simulink model "MicroGrid_Trifasico"  (R2017a)
settings: Solver=VariableStepAuto  StartTime=0.0  StopTime=.2  RelTol=1e-3
undefined symbols (not defined in the file or in its folder): st_time3
libraries: fl_lib x59, nesl_utility x25, powerlib_meascontrol x6, elec_lib x4
settings Model: Creator=erich  LastModifiedBy=erich

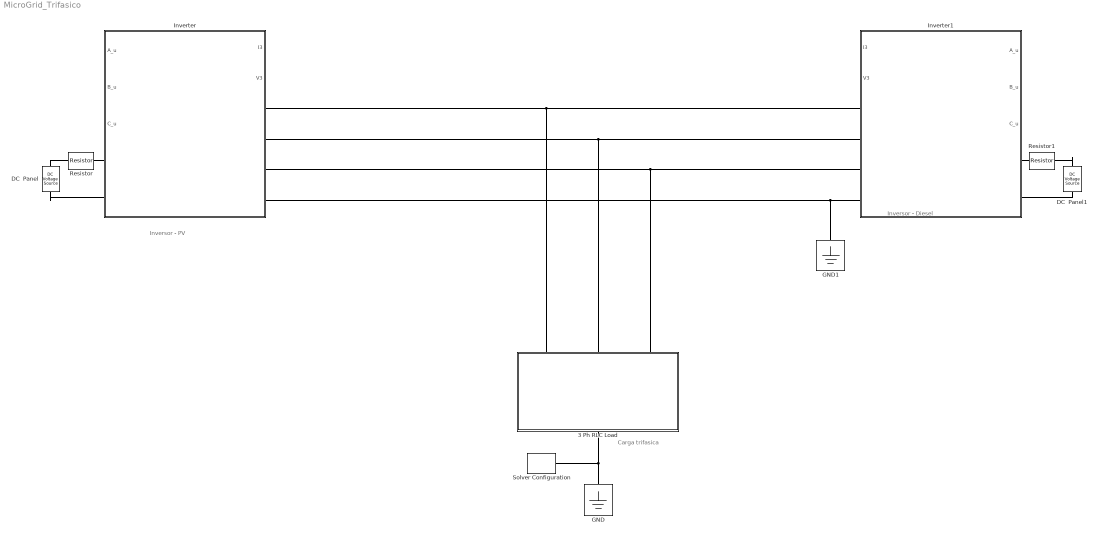
== system MicroGrid_Trifasico ==
  note: Carga trifasica
  note: Inversor - PV
  note: Inversor - Diesel
  3 Ph RLC Load : Subsystem
      mask Display:
      | port_label('lconn', 1, 'GND')
      | 
      | port_label('rconn', 1, 'Z_1', 'texmode', 'on')
      | port_label('rconn', 2, 'Z_2', 'texmode', 'on')
      | port_label('rconn', 3, 'Z_3', 'texmode', 'on')
      | 
      | plot([.15 .25], [.4 .4])
      | plot([.15 .25], [.48 .48])
      | plot([.20 .20], [.48 .6])
      | plot([.20 .20], [.4 .28])
      | 
      | plot(.43+abs(sin(200*[.2:.001:.5]/(2*pi))/15), [.2:.001:.5]+.1)
      | plot([.438 .438], [.2 .3])
      | plot([.438 .438], [.6 .7])
      | 
      | 
      | plot([.67 .73], [.6 .6])
      | plot([.67 .73], [.3 .3])
      | 
      | plot([.7 .7], [.2 .3])
      | plot([.7 .7], [.6 .7])
      | 
      | plot([.67 .67], [.6 .3])
      | plot([.73 .73], [.6 .3])
  DC  Panel : elec_lib/Additional Components/SPICE-Compatible Components/Sources/DC Voltage Source  DC=340 V
      settings: SourceProductName=Simscape Electronics  SourceProductBaseCode=SN
  DC  Panel1 : elec_lib/Additional Components/SPICE-Compatible Components/Sources/DC Voltage Source  DC=340 V
      settings: SourceProductName=Simscape Electronics  SourceProductBaseCode=SN
  GND : fl_lib/Electrical/Electrical Elements/Electrical Reference
  GND1 : fl_lib/Electrical/Electrical Elements/Electrical Reference
  Inverter : Subsystem
      mask Display:
      | port_label('input', 1, 'A_u')
      | port_label('input', 2, 'B_u')
      | port_label('input', 3, 'C_u')
      | 
      | port_label('lconn', 1, 'DC +')
      | port_label('lconn', 2, 'DC -')
      | 
      | 
      | port_label('rconn', 1, 'A')
      | port_label('rconn', 2, 'B')
      | port_label('rconn', 3, 'C')
      | 
      | port_label('output', 1, 'I_{3\Phi}', 'texmode', 'on')
      | port_label('output', 2, 'V_{3\Phi}', 'texmode', 'on')
      | 
      | plot([0.1 .9], [0.1 .9])
      | plot([0.2 .4], [.7 .7])
      | plot([0.2 .24], [.65 .65])
      | plot([0.28 .32], [.65 .65])
      | plot([0.36 .40], [.65 .65])
      | 
      | plot([.5:.01:.7], .25+sin(30*[.2:.01:.4])/10)
  Inverter1 : Subsystem
      mask Display:
      | port_label('input', 1, 'A_u')
      | port_label('input', 2, 'B_u')
      | port_label('input', 3, 'C_u')
      | 
      | port_label('lconn', 1, 'DC +')
      | port_label('lconn', 2, 'DC -')
      | 
      | 
      | port_label('rconn', 1, 'A')
      | port_label('rconn', 2, 'B')
      | port_label('rconn', 3, 'C')
      | 
      | port_label('output', 1, 'I_{3\Phi}', 'texmode', 'on')
      | port_label('output', 2, 'V_{3\Phi}', 'texmode', 'on')
      | 
      | plot([0.1 .9], [0.1 .9])
      | plot([0.2 .4], [.7 .7])
      | plot([0.2 .24], [.65 .65])
      | plot([0.28 .32], [.65 .65])
      | plot([0.36 .40], [.65 .65])
      | 
      | plot([.5:.01:.7], .25+sin(30*[.2:.01:.4])/10)
  Resistor : elec_lib/Passive Devices/Resistor  R=.01 Ohm  R_tol=5  enable_R_tol=0  tol_distribution=1  nSigma=4  enable_operating_limits=0  operating_limit_action=2  max_working_voltage=100 V  power_rating=1 W  enable_faults=0  fault_action=1  R_faulted=inf Ohm  enable_temporal_fault=0  t_fault=1 s  enable_behavioral_fault=0  max_permissible_current=1 A  t_fail_on_current=1 s  noise_mode=0  sample_time=1e-3 s  repeatability=1  auto_seed=1274213173  user_seed=0  Tdevice=25 degC  alpha=3.93e-3 1/K  Tmeas=25 degC  thermal_mass=100 J/K  power_derating_T1=70 degC  power_derating_T2=155 degC  operating_temperature_range_vec=[-50.0, 150.0] degC  temperature_specify=off  temperature_priority=High  temperature=298.15 K  temperature_nominal_specify=off  temperature_nominal_unit=K  temperature_nominal_value=1
  Resistor1 : elec_lib/Passive Devices/Resistor  R=1 Ohm  R_tol=5  enable_R_tol=0  tol_distribution=1  nSigma=4  enable_operating_limits=0  operating_limit_action=2  max_working_voltage=100 V  power_rating=1 W  enable_faults=0  fault_action=1  R_faulted=inf Ohm  enable_temporal_fault=0  t_fault=1 s  enable_behavioral_fault=0  max_permissible_current=1 A  t_fail_on_current=1 s  noise_mode=0  sample_time=1e-3 s  repeatability=1  auto_seed=306855934  user_seed=0  Tdevice=25 degC  alpha=3.93e-3 1/K  Tmeas=25 degC  thermal_mass=100 J/K  power_derating_T1=70 degC  power_derating_T2=155 degC  operating_temperature_range_vec=[-50.0, 150.0] degC  temperature_specify=off  temperature_priority=High  temperature=298.15 K  temperature_nominal_specify=off  temperature_nominal_unit=K  temperature_nominal_value=1
  Solver Configuration : nesl_utility/Solver Configuration  PhysicalDomain=network_engine_domain  SubClassName=solver  LeftPortType=input  RightPortType=generic  Accelerate=off  Tones=[]  Harmonics=[]  SimulateNoise=off  Profile=off  UseLocalSampling=off  EnableSwitchedLinearOptims=on  FrequencyDomain=off  UseCCode=off  RelTol=0.001  AbsTol=1e-06  MinStep=1e-09  ToWorkspace=off  RevertToSquareIcSolve=off  NumHomotopyIterations=100  PhasorMode=off  PhasorModeNumHarmonics=1  OverrideAbsTol=off  DoDC=off  ResidualTolerance=1e-09  UseLocalSolver=on  LocalSolverChoice=NE_BACKWARD_EULER_ADVANCER  LocalSolverSampleTime=1e-6  DoFixedCost=on  MaxNonlinIter=3  MaxModeIter=2  LinearAlgebra=Sparse  DelaysMemoryBudget=1024  AutomaticFiltering=on  FilteringTimeConstant=0.001
  connections:
  3 Ph RLC Load/LConn1 -- GND/LConn1 -- Solver Configuration/RConn1
  Resistor/LConn1 -- DC  Panel/LConn1
  DC  Panel/RConn1 -- Inverter/LConn2
  Resistor/RConn1 -- Inverter/LConn1
  Inverter1/LConn2 -- DC  Panel1/LConn1
  DC  Panel1/RConn1 -- Resistor1/LConn1
  Inverter1/LConn1 -- Resistor1/RConn1
  Inverter/RConn1 -- 3 Ph RLC Load/RConn1 -- Inverter1/RConn1
  Inverter1/RConn2 -- 3 Ph RLC Load/RConn2 -- Inverter/RConn2
  Inverter1/RConn3 -- 3 Ph RLC Load/RConn3 -- Inverter/RConn3
  Inverter1/RConn4 -- GND1/LConn1 -- Inverter/RConn4

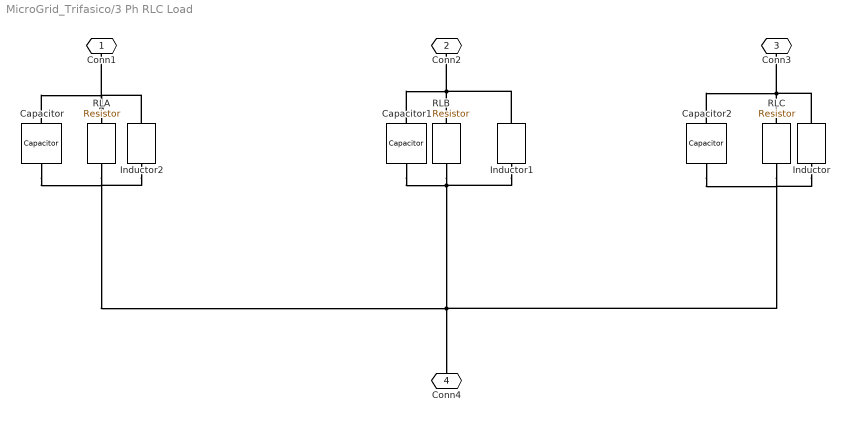
== system MicroGrid_Trifasico/3 Ph RLC Load ==
  Capacitor : fl_lib/Electrical/Electrical Elements/Capacitor  c=100e-6 uF  r=1e-6 Ohm  g=0 1/Ohm  i_specify=off  i_priority=None  i=0 A  i_nominal_specify=off  i_nominal_unit=A  i_nominal_value=1  v_specify=off  v_priority=None  v=0 V  v_nominal_specify=off  v_nominal_unit=V  v_nominal_value=1  vc_specify=off  vc_priority=High  vc=0 V  vc_nominal_specify=off  vc_nominal_unit=V  vc_nominal_value=1
  Capacitor1 : fl_lib/Electrical/Electrical Elements/Capacitor  c=100e-6 uF  r=1e-6 Ohm  g=0 1/Ohm  i_specify=off  i_priority=None  i=0 A  i_nominal_specify=off  i_nominal_unit=A  i_nominal_value=1  v_specify=off  v_priority=None  v=0 V  v_nominal_specify=off  v_nominal_unit=V  v_nominal_value=1  vc_specify=off  vc_priority=High  vc=0 V  vc_nominal_specify=off  vc_nominal_unit=V  vc_nominal_value=1
  Capacitor2 : fl_lib/Electrical/Electrical Elements/Capacitor  c=100e-6 uF  r=1e-6 Ohm  g=0 1/Ohm  i_specify=off  i_priority=None  i=0 A  i_nominal_specify=off  i_nominal_unit=A  i_nominal_value=1  v_specify=off  v_priority=None  v=0 V  v_nominal_specify=off  v_nominal_unit=V  v_nominal_value=1  vc_specify=off  vc_priority=High  vc=0 V  vc_nominal_specify=off  vc_nominal_unit=V  vc_nominal_value=1
  Inductor : fl_lib/Electrical/Electrical Elements/Inductor  l=5200 mH  r=0 Ohm  g=100e-9 1/Ohm  i_specify=off  i_priority=None  i=0 A  i_nominal_specify=off  i_nominal_unit=A  i_nominal_value=1  v_specify=off  v_priority=None  v=0 V  v_nominal_specify=off  v_nominal_unit=V  v_nominal_value=1  i_L_specify=off  i_L_priority=High  i_L=0 A  i_L_nominal_specify=off  i_L_nominal_unit=A  i_L_nominal_value=1
  Inductor1 : fl_lib/Electrical/Electrical Elements/Inductor  l=5200 mH  r=0 Ohm  g=100e-9 1/Ohm  i_specify=off  i_priority=None  i=0 A  i_nominal_specify=off  i_nominal_unit=A  i_nominal_value=1  v_specify=off  v_priority=None  v=0 V  v_nominal_specify=off  v_nominal_unit=V  v_nominal_value=1  i_L_specify=off  i_L_priority=High  i_L=0 A  i_L_nominal_specify=off  i_L_nominal_unit=A  i_L_nominal_value=1
  Inductor2 : fl_lib/Electrical/Electrical Elements/Inductor  l=5200 mH  r=0 Ohm  g=100e-9 1/Ohm  i_specify=off  i_priority=None  i=0 A  i_nominal_specify=off  i_nominal_unit=A  i_nominal_value=1  v_specify=off  v_priority=None  v=0 V  v_nominal_specify=off  v_nominal_unit=V  v_nominal_value=1  i_L_specify=off  i_L_priority=High  i_L=0 A  i_L_nominal_specify=off  i_L_nominal_unit=A  i_L_nominal_value=1
  RLA : fl_lib/Electrical/Electrical Elements/Resistor  R=15 Ohm  i_specify=off  i_priority=None  i=0 A  i_nominal_specify=off  i_nominal_unit=A  i_nominal_value=1  v_specify=off  v_priority=None  v=0 V  v_nominal_specify=off  v_nominal_unit=V  v_nominal_value=1
  RLB : fl_lib/Electrical/Electrical Elements/Resistor  R=15 Ohm  i_specify=off  i_priority=None  i=0 A  i_nominal_specify=off  i_nominal_unit=A  i_nominal_value=1  v_specify=off  v_priority=None  v=0 V  v_nominal_specify=off  v_nominal_unit=V  v_nominal_value=1
  RLC : fl_lib/Electrical/Electrical Elements/Resistor  R=15 Ohm  i_specify=off  i_priority=None  i=0 A  i_nominal_specify=off  i_nominal_unit=A  i_nominal_value=1  v_specify=off  v_priority=None  v=0 V  v_nominal_specify=off  v_nominal_unit=V  v_nominal_value=1
  Conn1 : PMIOPort  Port=1  Side=Right
  Conn2 : PMIOPort  Port=2  Side=Right
  Conn3 : PMIOPort  Port=3  Side=Right
  Conn4 : PMIOPort  Port=4  Side=Left
  connections:
  RLB/RConn1 -- Capacitor1/RConn1 -- Inductor1/RConn1 -- Conn4/RConn1 -- Inductor2/RConn1 -- Capacitor/RConn1 -- RLA/RConn1 -- Capacitor2/RConn1 -- Inductor/RConn1 -- RLC/RConn1
  RLA/LConn1 -- Inductor2/LConn1 -- Conn1/RConn1 -- Capacitor/LConn1
  RLC/LConn1 -- Capacitor2/LConn1 -- Conn3/RConn1 -- Inductor/LConn1
  RLB/LConn1 -- Conn2/RConn1 -- Capacitor1/LConn1 -- Inductor1/LConn1

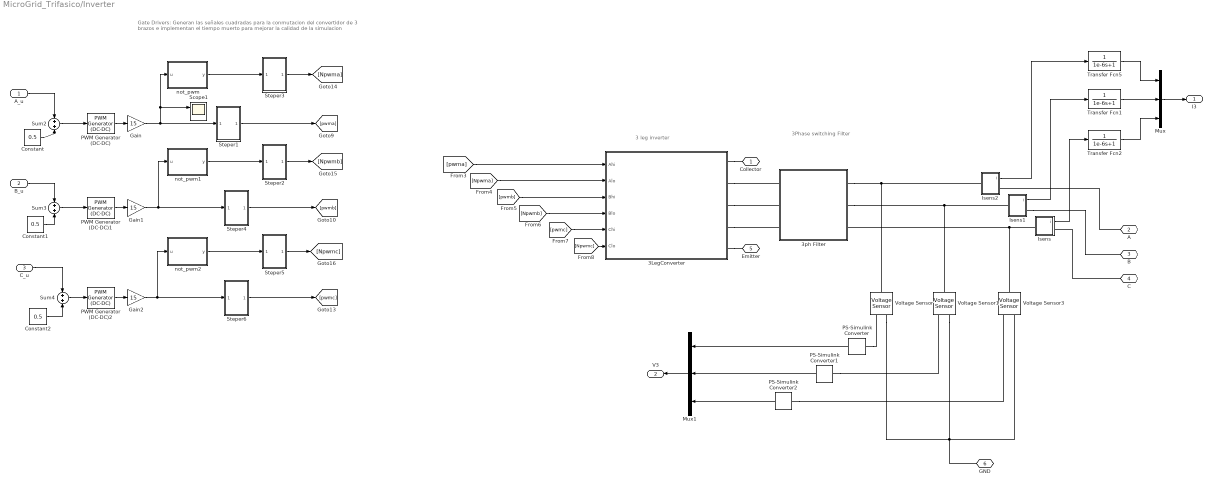
== system MicroGrid_Trifasico/Inverter ==
  note: Gate Drivers: Generan las señales cuadradas para
      | la conmutacion del convertidor de 3 brazos e implementan el
      | tiempo muerto para mejorar la calidad de la simulacion
  note: 3 leg inverter
  note: 3Phase
      | switching
      | Filter
  A_u : Inport
  B_u : Inport  Port=2
  C_u : Inport  Port=3
  3LegConverter : Subsystem
      mask Display:
      | % entradas de conmutacion del mosfet
      | port_label('input',1,'Ahi')
      | port_label('input',2,'Alo')
      | port_label('input',3,'Bhi')
      | port_label('input',4,'Blo')
      | port_label('input',5,'Chi')
      | port_label('input',6,'Clo')
      | 
      | % puertos de conexion del inversor
      | port_label('rconn',1,'Collector') % + fuente dc
      | port_label('rconn',2,'A') % fase A
      | port_label('rconn',3,'B') % fase B
      | port_label('rconn',4,'C') % fase C
      | port_label('rconn',5,'Emitter') % ref fuente dc
      | 
      | 
      | plot([.4 .4],[.35 .7])
      | plot([.2 .4],[.52 .52])
      | plot([.46 .46],[.22 .85])
      | plot([.46 .7],[.73 .73])
      | plot([.46 .7],[.32 .32])
  3ph Filter : Subsystem
      mask Display:
      | port_label('lconn', 1, 'A_{in}', 'texmode', 'on')
      | port_label('lconn', 2, 'B_{in}', 'texmode', 'on')
      | port_label('lconn', 3, 'B_{in}', 'texmode', 'on')
      | port_label('rconn', 1, 'A_{out}', 'texmode', 'on')
      | port_label('rconn', 2, 'B_{out}', 'texmode', 'on')
      | port_label('rconn', 3, 'C_{out}', 'texmode', 'on')
      | 
      | 
      | plot([.2 .5], [.7 .7])
      | plot([.5 .6], [.7 .3])
      | plot([.6 .7], [.3 .3])
      | 
      | text(.2, .8, '\fontsize{12} H(\omega)', 'texmode', 'on')
      | text(.6, .25, '\fontsize{12} \omega', 'texmode', 'on')
  Constant : Constant  Value=0.5
  Constant1 : Constant  Value=0.5
  Constant2 : Constant  Value=0.5
  Gain : Gain  Gain=15
  Gain1 : Gain  Gain=15
  Gain2 : Gain  Gain=15
  Isens : Subsystem
  Isens1 : Subsystem
  Isens2 : Subsystem
  Mux : Mux  Inputs=3
  Mux1 : Mux  Inputs=3
  PS-Simulink Converter : nesl_utility/PS-Simulink Converter  PhysicalDomain=network_engine_domain  SubClassName=ps_output  LeftPortType=input  RightPortType=output  PseudoPeriodic=off  Frequencies=[]  Unit=1  AffineConversion=off
  PS-Simulink Converter1 : nesl_utility/PS-Simulink Converter  PhysicalDomain=network_engine_domain  SubClassName=ps_output  LeftPortType=input  RightPortType=output  PseudoPeriodic=off  Frequencies=[]  Unit=1  AffineConversion=off
  PS-Simulink Converter2 : nesl_utility/PS-Simulink Converter  PhysicalDomain=network_engine_domain  SubClassName=ps_output  LeftPortType=input  RightPortType=output  PseudoPeriodic=off  Frequencies=[]  Unit=1  AffineConversion=off
  PWM Generator (DC-DC) : powerlib_meascontrol/Pulse & Signal Generators/PWM Generator (DC-DC)  Fsw=5000  Ts=0
  PWM Generator (DC-DC)1 : powerlib_meascontrol/Pulse & Signal Generators/PWM Generator (DC-DC)  Fsw=5000  Ts=0
  PWM Generator (DC-DC)2 : powerlib_meascontrol/Pulse & Signal Generators/PWM Generator (DC-DC)  Fsw=5000  Ts=0
  Scope1 : Scope  NumInputPorts=2
  Steper1 : Subsystem
  Steper2 : Subsystem
  Steper3 : Subsystem
  Steper4 : Subsystem
  Steper5 : Subsystem
  Steper6 : Subsystem
  Sum2 : Sum
  Sum3 : Sum
  Sum4 : Sum
  Transfer Fcn1 : TransferFcn  Denominator=[1e-6 1]
  Transfer Fcn2 : TransferFcn  Denominator=[1e-6 1]
  Transfer Fcn5 : TransferFcn  Denominator=[1e-6 1]
  Voltage Sensor : fl_lib/Electrical/Electrical Sensors/Voltage Sensor
  Voltage Sensor1 : fl_lib/Electrical/Electrical Sensors/Voltage Sensor
  Voltage Sensor3 : fl_lib/Electrical/Electrical Sensors/Voltage Sensor
  not_pwm : MATLAB Function  TreatAsAtomicUnit=on
  not_pwm1 : MATLAB Function  TreatAsAtomicUnit=on
  not_pwm2 : MATLAB Function  TreatAsAtomicUnit=on
  Collector : PMIOPort  Port=1  Side=Left
  A : PMIOPort  Port=2  Side=Right
  B : PMIOPort  Port=3  Side=Right
  C : PMIOPort  Port=4  Side=Right
  Emitter : PMIOPort  Port=5  Side=Left
  GND : PMIOPort  Port=6  Side=Right
  I3 : Outport
  V3 : Outport  Port=2
  wires:
  C_u/1 -> Sum4/1
  [Npwmc] -> 3LegConverter/6(Clo)
  [pwma] -> 3LegConverter/1(Ahi)
  [pwmc] -> 3LegConverter/5(Chi)
  [Npwma] -> 3LegConverter/2(Alo)
  [Npwmb] -> 3LegConverter/4(Blo)
  [pwmb] -> 3LegConverter/3(Bhi)
  Steper5/1(Out1) -> [Npwmc]
  Steper4/1(Out1) -> [pwmb]
  Gain/1 -> Steper1/1(In1), Scope1/1, not_pwm/1(u)
  not_pwm1/1(y) -> Steper2/1(In1)
  Steper3/1(Out1) -> [Npwma]
  Constant/1 -> Sum2/2
  Sum2/1 -> PWM Generator (DC-DC)/1
  Gain2/1 -> Steper6/1(In1), not_pwm2/1(u)
  Sum3/1 -> PWM Generator (DC-DC)1/1
  Steper6/1(Out1) -> [pwmc]
  Sum4/1 -> PWM Generator (DC-DC)2/1
  Gain1/1 -> Steper4/1(In1), not_pwm1/1(u)
  not_pwm2/1(y) -> Steper5/1(In1)
  Steper2/1(Out1) -> [Npwmb]
  Constant2/1 -> Sum4/2
  PWM Generator (DC-DC)1/1 -> Gain1/1
  not_pwm/1(y) -> Steper3/1(In1)
  PWM Generator (DC-DC)/1 -> Gain/1
  PWM Generator (DC-DC)2/1 -> Gain2/1
  Steper1/1(Out1) -> [pwma]
  Constant1/1 -> Sum3/2
  B_u/1 -> Sum3/1
  A_u/1 -> Sum2/1
  Isens/1(i) -> Transfer Fcn2/1
  Isens1/1(i) -> Transfer Fcn1/1
  Isens2/1(i) -> Transfer Fcn5/1
  Mux/1 -> I3/1
  Transfer Fcn1/1 -> Mux/2
  Transfer Fcn5/1 -> Mux/1
  Transfer Fcn2/1 -> Mux/3
  Mux1/1 -> V3/1
  PS-Simulink Converter/1 -> Mux1/1
  PS-Simulink Converter1/1 -> Mux1/2
  PS-Simulink Converter2/1 -> Mux1/3
  connections:
  3LegConverter/RConn5 -- Emitter/RConn1
  3LegConverter/RConn1 -- Collector/RConn1
  C/RConn1 -- Isens/RConn1
  Isens1/RConn1 -- B/RConn1
  A/RConn1 -- Isens2/RConn1
  3LegConverter/RConn2 -- 3ph Filter/LConn1
  3LegConverter/RConn3 -- 3ph Filter/LConn2
  3LegConverter/RConn4 -- 3ph Filter/LConn3
  3ph Filter/RConn1 -- Voltage Sensor/LConn1 -- Isens2/LConn1
  3ph Filter/RConn2 -- Isens1/LConn1 -- Voltage Sensor1/LConn1
  Isens/LConn1 -- Voltage Sensor3/LConn1 -- 3ph Filter/RConn3
  Voltage Sensor1/RConn2 -- Voltage Sensor3/RConn2 -- GND/RConn1 -- Voltage Sensor/RConn2
  PS-Simulink Converter1/LConn1 -- Voltage Sensor1/RConn1
  PS-Simulink Converter2/LConn1 -- Voltage Sensor3/RConn1
  PS-Simulink Converter/LConn1 -- Voltage Sensor/RConn1

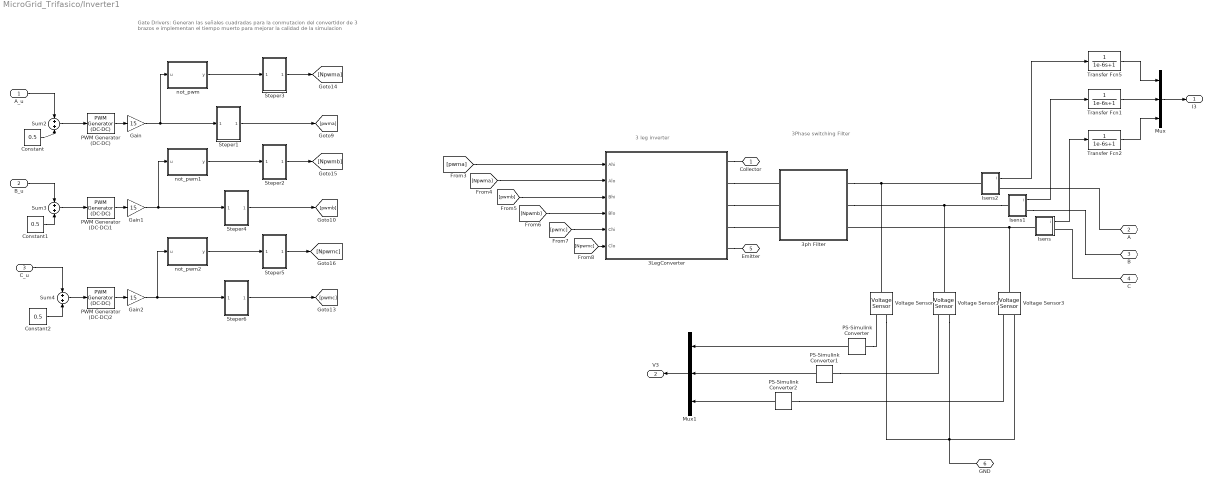
== system MicroGrid_Trifasico/Inverter1 ==
  note: 3Phase
      | switching
      | Filter
  note: 3 leg inverter
  note: Gate Drivers: Generan las señales cuadradas para
      | la conmutacion del convertidor de 3 brazos e implementan el
      | tiempo muerto para mejorar la calidad de la simulacion
  A_u : Inport
  B_u : Inport  Port=2
  C_u : Inport  Port=3
  3LegConverter : Subsystem
      mask Display:
      | % entradas de conmutacion del mosfet
      | port_label('input',1,'Ahi')
      | port_label('input',2,'Alo')
      | port_label('input',3,'Bhi')
      | port_label('input',4,'Blo')
      | port_label('input',5,'Chi')
      | port_label('input',6,'Clo')
      | 
      | % puertos de conexion del inversor
      | port_label('rconn',1,'Collector') % + fuente dc
      | port_label('rconn',2,'A') % fase A
      | port_label('rconn',3,'B') % fase B
      | port_label('rconn',4,'C') % fase C
      | port_label('rconn',5,'Emitter') % ref fuente dc
      | 
      | 
      | plot([.4 .4],[.35 .7])
      | plot([.2 .4],[.52 .52])
      | plot([.46 .46],[.22 .85])
      | plot([.46 .7],[.73 .73])
      | plot([.46 .7],[.32 .32])
  3ph Filter : Subsystem
  Constant : Constant  Value=0.5
  Constant1 : Constant  Value=0.5
  Constant2 : Constant  Value=0.5
  Gain : Gain  Gain=15
  Gain1 : Gain  Gain=15
  Gain2 : Gain  Gain=15
  Isens : Subsystem
  Isens1 : Subsystem
  Isens2 : Subsystem
  Mux : Mux  Inputs=3
  Mux1 : Mux  Inputs=3
  PS-Simulink Converter : nesl_utility/PS-Simulink Converter  PhysicalDomain=network_engine_domain  SubClassName=ps_output  LeftPortType=input  RightPortType=output  PseudoPeriodic=off  Frequencies=[]  Unit=1  AffineConversion=off
  PS-Simulink Converter1 : nesl_utility/PS-Simulink Converter  PhysicalDomain=network_engine_domain  SubClassName=ps_output  LeftPortType=input  RightPortType=output  PseudoPeriodic=off  Frequencies=[]  Unit=1  AffineConversion=off
  PS-Simulink Converter2 : nesl_utility/PS-Simulink Converter  PhysicalDomain=network_engine_domain  SubClassName=ps_output  LeftPortType=input  RightPortType=output  PseudoPeriodic=off  Frequencies=[]  Unit=1  AffineConversion=off
  PWM Generator (DC-DC) : powerlib_meascontrol/Pulse & Signal Generators/PWM Generator (DC-DC)  Fsw=5000  Ts=0
  PWM Generator (DC-DC)1 : powerlib_meascontrol/Pulse & Signal Generators/PWM Generator (DC-DC)  Fsw=5000  Ts=0
  PWM Generator (DC-DC)2 : powerlib_meascontrol/Pulse & Signal Generators/PWM Generator (DC-DC)  Fsw=5000  Ts=0
  Steper1 : Subsystem
  Steper2 : Subsystem
  Steper3 : Subsystem
  Steper4 : Subsystem
  Steper5 : Subsystem
  Steper6 : Subsystem
  Sum2 : Sum
  Sum3 : Sum
  Sum4 : Sum
  Transfer Fcn1 : TransferFcn  Denominator=[1e-6 1]
  Transfer Fcn2 : TransferFcn  Denominator=[1e-6 1]
  Transfer Fcn5 : TransferFcn  Denominator=[1e-6 1]
  Voltage Sensor : fl_lib/Electrical/Electrical Sensors/Voltage Sensor
  Voltage Sensor1 : fl_lib/Electrical/Electrical Sensors/Voltage Sensor
  Voltage Sensor3 : fl_lib/Electrical/Electrical Sensors/Voltage Sensor
  not_pwm : MATLAB Function  TreatAsAtomicUnit=on
  not_pwm1 : MATLAB Function  TreatAsAtomicUnit=on
  not_pwm2 : MATLAB Function  TreatAsAtomicUnit=on
  Collector : PMIOPort  Port=1  Side=Left
  A : PMIOPort  Port=2  Side=Right
  B : PMIOPort  Port=3  Side=Right
  C : PMIOPort  Port=4  Side=Right
  Emitter : PMIOPort  Port=5  Side=Left
  GND : PMIOPort  Port=6  Side=Right
  I3 : Outport
  V3 : Outport  Port=2
  wires:
  PS-Simulink Converter2/1 -> Mux1/3
  PS-Simulink Converter1/1 -> Mux1/2
  PS-Simulink Converter/1 -> Mux1/1
  Mux1/1 -> V3/1
  Transfer Fcn2/1 -> Mux/3
  Transfer Fcn5/1 -> Mux/1
  Transfer Fcn1/1 -> Mux/2
  Mux/1 -> I3/1
  Isens2/1(i) -> Transfer Fcn5/1
  Isens1/1(i) -> Transfer Fcn1/1
  Isens/1(i) -> Transfer Fcn2/1
  A_u/1 -> Sum2/1
  B_u/1 -> Sum3/1
  Constant1/1 -> Sum3/2
  Steper1/1(Out1) -> [pwma]
  PWM Generator (DC-DC)2/1 -> Gain2/1
  PWM Generator (DC-DC)/1 -> Gain/1
  not_pwm/1(y) -> Steper3/1(In1)
  PWM Generator (DC-DC)1/1 -> Gain1/1
  Constant2/1 -> Sum4/2
  Steper2/1(Out1) -> [Npwmb]
  not_pwm2/1(y) -> Steper5/1(In1)
  Gain1/1 -> not_pwm1/1(u), Steper4/1(In1)
  Sum4/1 -> PWM Generator (DC-DC)2/1
  Steper6/1(Out1) -> [pwmc]
  Sum3/1 -> PWM Generator (DC-DC)1/1
  Gain2/1 -> not_pwm2/1(u), Steper6/1(In1)
  Sum2/1 -> PWM Generator (DC-DC)/1
  Constant/1 -> Sum2/2
  Steper3/1(Out1) -> [Npwma]
  not_pwm1/1(y) -> Steper2/1(In1)
  Gain/1 -> not_pwm/1(u), Steper1/1(In1)
  Steper4/1(Out1) -> [pwmb]
  Steper5/1(Out1) -> [Npwmc]
  [pwmb] -> 3LegConverter/3(Bhi)
  [Npwmb] -> 3LegConverter/4(Blo)
  [Npwma] -> 3LegConverter/2(Alo)
  [pwmc] -> 3LegConverter/5(Chi)
  [pwma] -> 3LegConverter/1(Ahi)
  [Npwmc] -> 3LegConverter/6(Clo)
  C_u/1 -> Sum4/1
  connections:
  PS-Simulink Converter/LConn1 -- Voltage Sensor/RConn1
  PS-Simulink Converter2/LConn1 -- Voltage Sensor3/RConn1
  PS-Simulink Converter1/LConn1 -- Voltage Sensor1/RConn1
  Voltage Sensor3/RConn2 -- Voltage Sensor/RConn2 -- GND/RConn1 -- Voltage Sensor1/RConn2
  Voltage Sensor3/LConn1 -- 3ph Filter/RConn3 -- Isens/LConn1
  Isens1/LConn1 -- 3ph Filter/RConn2 -- Voltage Sensor1/LConn1
  Voltage Sensor/LConn1 -- 3ph Filter/RConn1 -- Isens2/LConn1
  3LegConverter/RConn4 -- 3ph Filter/LConn3
  3LegConverter/RConn3 -- 3ph Filter/LConn2
  3LegConverter/RConn2 -- 3ph Filter/LConn1
  A/RConn1 -- Isens2/RConn1
  Isens1/RConn1 -- B/RConn1
  C/RConn1 -- Isens/RConn1
  3LegConverter/RConn1 -- Collector/RConn1
  3LegConverter/RConn5 -- Emitter/RConn1

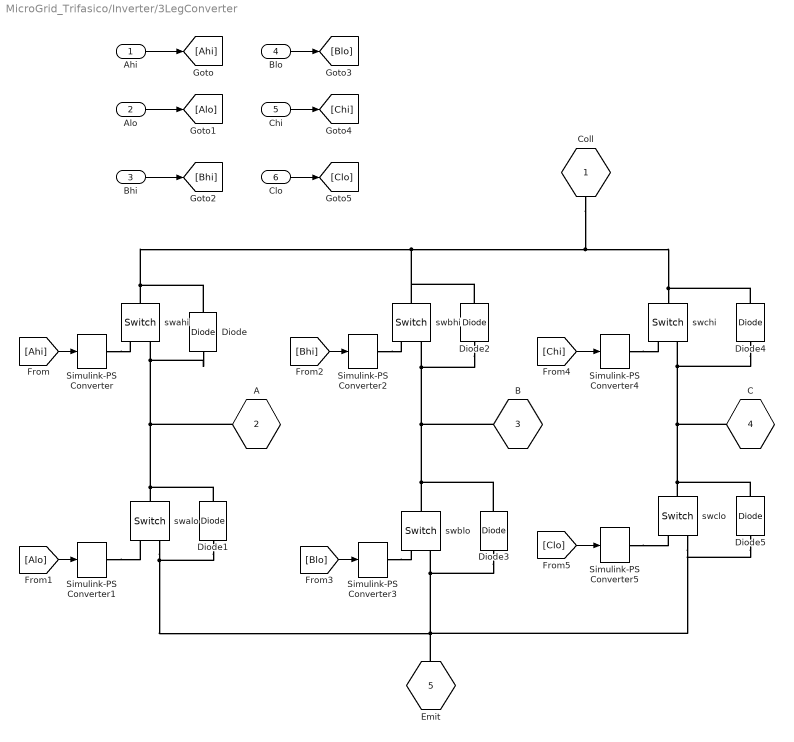
== system MicroGrid_Trifasico/Inverter/3LegConverter ==
  Ahi : Inport
  Alo : Inport  Port=2
  Bhi : Inport  Port=3
  Blo : Inport  Port=4
  Chi : Inport  Port=5
  Clo : Inport  Port=6
  Diode{,1..5} (6 alike) : fl_lib/Electrical/Electrical Elements/Diode  Vf=0.6 V  Ron=0.3 Ohm  Goff=1e-8 1/Ohm  i_specify=off  i_priority=None  i=0 A  i_nominal_specify=off  i_nominal_unit=A  i_nominal_value=1  v_specify=off  v_priority=None  v=0 V  v_nominal_specify=off  v_nominal_unit=V  v_nominal_value=1
  Simulink-PS Converter{,1..5} (6 alike) : nesl_utility/Simulink-PS Converter  PhysicalDomain=network_engine_domain  SubClassName=ps_input  LeftPortType=input  RightPortType=output  PseudoPeriodic=off  Frequencies=[]  NoiseDistribution=none  NoiseParameters=[]  Unit=1  AffineConversion=off  FilteringAndDerivatives=zero  SimscapeFilterOrder=1  InputFilterTimeConstant=0.001  UdotUserProvided=1
  swahi : fl_lib/Electrical/Electrical Elements/Switch  R_closed=0.01 Ohm  G_open=1e-8 1/Ohm  Threshold=2  i_specify=off  i_priority=None  i=0 A  i_nominal_specify=off  i_nominal_unit=A  i_nominal_value=1  v_specify=off  v_priority=None  v=0 V  v_nominal_specify=off  v_nominal_unit=V  v_nominal_value=1
      settings: SourceProductName=Simscape
  swalo : fl_lib/Electrical/Electrical Elements/Switch  R_closed=0.01 Ohm  G_open=1e-8 1/Ohm  Threshold=2  i_specify=off  i_priority=None  i=0 A  i_nominal_specify=off  i_nominal_unit=A  i_nominal_value=1  v_specify=off  v_priority=None  v=0 V  v_nominal_specify=off  v_nominal_unit=V  v_nominal_value=1
      settings: SourceProductName=Simscape
  swbhi : fl_lib/Electrical/Electrical Elements/Switch  R_closed=0.01 Ohm  G_open=1e-8 1/Ohm  Threshold=2  i_specify=off  i_priority=None  i=0 A  i_nominal_specify=off  i_nominal_unit=A  i_nominal_value=1  v_specify=off  v_priority=None  v=0 V  v_nominal_specify=off  v_nominal_unit=V  v_nominal_value=1
      settings: SourceProductName=Simscape
  swblo : fl_lib/Electrical/Electrical Elements/Switch  R_closed=0.01 Ohm  G_open=1e-8 1/Ohm  Threshold=2  i_specify=off  i_priority=None  i=0 A  i_nominal_specify=off  i_nominal_unit=A  i_nominal_value=1  v_specify=off  v_priority=None  v=0 V  v_nominal_specify=off  v_nominal_unit=V  v_nominal_value=1
      settings: SourceProductName=Simscape
  swchi : fl_lib/Electrical/Electrical Elements/Switch  R_closed=0.01 Ohm  G_open=1e-8 1/Ohm  Threshold=2  i_specify=off  i_priority=None  i=0 A  i_nominal_specify=off  i_nominal_unit=A  i_nominal_value=1  v_specify=off  v_priority=None  v=0 V  v_nominal_specify=off  v_nominal_unit=V  v_nominal_value=1
      settings: SourceProductName=Simscape
  swclo : fl_lib/Electrical/Electrical Elements/Switch  R_closed=0.01 Ohm  G_open=1e-8 1/Ohm  Threshold=2  i_specify=off  i_priority=None  i=0 A  i_nominal_specify=off  i_nominal_unit=A  i_nominal_value=1  v_specify=off  v_priority=None  v=0 V  v_nominal_specify=off  v_nominal_unit=V  v_nominal_value=1
      settings: SourceProductName=Simscape
  Coll : PMIOPort  Port=1  Side=Right
  A : PMIOPort  Port=2  Side=Right
  B : PMIOPort  Port=3  Side=Right
  C : PMIOPort  Port=4  Side=Right
  Emit : PMIOPort  Port=5  Side=Right
  wires:
  [Alo] -> Simulink-PS Converter1/1
  [Ahi] -> Simulink-PS Converter/1
  Clo/1 -> [Clo]
  Alo/1 -> [Alo]
  [Blo] -> Simulink-PS Converter3/1
  [Clo] -> Simulink-PS Converter5/1
  Bhi/1 -> [Bhi]
  [Bhi] -> Simulink-PS Converter2/1
  Ahi/1 -> [Ahi]
  [Chi] -> Simulink-PS Converter4/1
  Blo/1 -> [Blo]
  Chi/1 -> [Chi]
  connections:
  swalo/RConn2 -- Diode3/LConn1 -- swblo/RConn2 -- Emit/RConn1 -- Diode5/LConn1 -- swclo/RConn2 -- Diode1/LConn1
  Simulink-PS Converter4/RConn1 -- swchi/RConn1
  Simulink-PS Converter5/RConn1 -- swclo/RConn1
  Simulink-PS Converter/RConn1 -- swahi/RConn1
  swblo/LConn1 -- Diode3/RConn1 -- B/RConn1 -- Diode2/LConn1 -- swbhi/RConn2
  Simulink-PS Converter3/RConn1 -- swblo/RConn1
  Simulink-PS Converter2/RConn1 -- swbhi/RConn1
  Simulink-PS Converter1/RConn1 -- swalo/RConn1
  swalo/LConn1 -- A/RConn1 -- Diode/LConn1 -- swahi/RConn2 -- Diode1/RConn1
  swahi/LConn1 -- Diode/RConn1 -- Diode2/RConn1 -- swbhi/LConn1 -- Coll/RConn1 -- Diode4/RConn1 -- swchi/LConn1
  swclo/LConn1 -- Diode5/RConn1 -- C/RConn1 -- Diode4/LConn1 -- swchi/RConn2

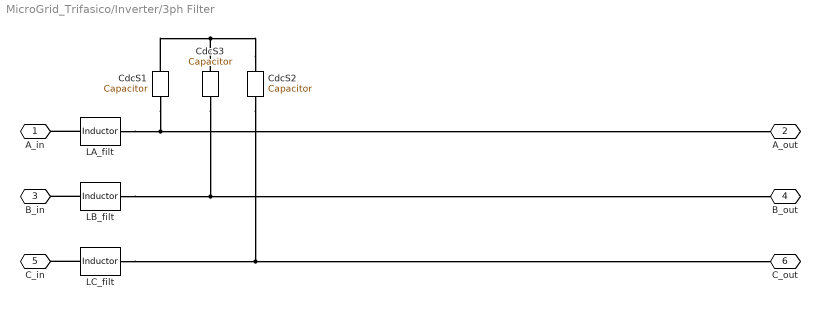
== system MicroGrid_Trifasico/Inverter/3ph Filter ==
  CdcS1 : fl_lib/Electrical/Electrical Elements/Capacitor  c=3.5 uF  r=1e-6 Ohm  g=0 1/Ohm  i_specify=off  i_priority=None  i=0 A  i_nominal_specify=off  i_nominal_unit=A  i_nominal_value=1  v_specify=off  v_priority=None  v=0 V  v_nominal_specify=off  v_nominal_unit=V  v_nominal_value=1  vc_specify=on  vc_priority=High  vc=0 V  vc_nominal_specify=off  vc_nominal_unit=V  vc_nominal_value=1
  CdcS2 : fl_lib/Electrical/Electrical Elements/Capacitor  c=3.5 uF  r=1e-6 Ohm  g=0 1/Ohm  i_specify=off  i_priority=None  i=0 A  i_nominal_specify=off  i_nominal_unit=A  i_nominal_value=1  v_specify=off  v_priority=None  v=0 V  v_nominal_specify=off  v_nominal_unit=V  v_nominal_value=1  vc_specify=on  vc_priority=High  vc=0 V  vc_nominal_specify=off  vc_nominal_unit=V  vc_nominal_value=1
  CdcS3 : fl_lib/Electrical/Electrical Elements/Capacitor  c=3.5 uF  r=1e-6 Ohm  g=0 1/Ohm  i_specify=off  i_priority=None  i=0 A  i_nominal_specify=off  i_nominal_unit=A  i_nominal_value=1  v_specify=off  v_priority=None  v=0 V  v_nominal_specify=off  v_nominal_unit=V  v_nominal_value=1  vc_specify=on  vc_priority=High  vc=0 V  vc_nominal_specify=off  vc_nominal_unit=V  vc_nominal_value=1
  LA_filt : fl_lib/Electrical/Electrical Elements/Inductor  l=6.2 mH  r=0.1 Ohm  g=1e-6 1/Ohm  i_specify=off  i_priority=None  i=0 A  i_nominal_specify=off  i_nominal_unit=A  i_nominal_value=1  v_specify=off  v_priority=None  v=0 V  v_nominal_specify=off  v_nominal_unit=V  v_nominal_value=1  i_L_specify=on  i_L_priority=High  i_L=0 A  i_L_nominal_specify=off  i_L_nominal_unit=A  i_L_nominal_value=1
  LB_filt : fl_lib/Electrical/Electrical Elements/Inductor  l=6.2 mH  r=2 Ohm  g=1e-6 1/Ohm  i_specify=off  i_priority=None  i=0 A  i_nominal_specify=off  i_nominal_unit=A  i_nominal_value=1  v_specify=off  v_priority=None  v=0 V  v_nominal_specify=off  v_nominal_unit=V  v_nominal_value=1  i_L_specify=on  i_L_priority=High  i_L=0 A  i_L_nominal_specify=off  i_L_nominal_unit=A  i_L_nominal_value=1
  LC_filt : fl_lib/Electrical/Electrical Elements/Inductor  l=6.2 mH  r=2 Ohm  g=1e-6 1/Ohm  i_specify=off  i_priority=None  i=0 A  i_nominal_specify=off  i_nominal_unit=A  i_nominal_value=1  v_specify=off  v_priority=None  v=0 V  v_nominal_specify=off  v_nominal_unit=V  v_nominal_value=1  i_L_specify=on  i_L_priority=High  i_L=0 A  i_L_nominal_specify=off  i_L_nominal_unit=A  i_L_nominal_value=1
  A_in : PMIOPort  Port=1  Side=Left
  A_out : PMIOPort  Port=2  Side=Right
  B_in : PMIOPort  Port=3  Side=Left
  B_out : PMIOPort  Port=4  Side=Right
  C_in : PMIOPort  Port=5  Side=Left
  C_out : PMIOPort  Port=6  Side=Right
  connections:
  CdcS1/RConn1 -- A_out/RConn1 -- LA_filt/RConn1
  CdcS2/LConn1 -- CdcS1/LConn1 -- CdcS3/LConn1
  CdcS3/RConn1 -- B_out/RConn1 -- LB_filt/RConn1
  CdcS2/RConn1 -- C_out/RConn1 -- LC_filt/RConn1
  LC_filt/LConn1 -- C_in/RConn1
  LA_filt/LConn1 -- A_in/RConn1
  LB_filt/LConn1 -- B_in/RConn1

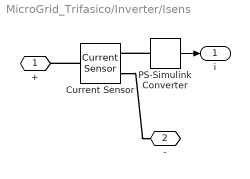
== system MicroGrid_Trifasico/Inverter/Isens ==
  Current Sensor : fl_lib/Electrical/Electrical Sensors/Current Sensor
  PS-Simulink Converter : nesl_utility/PS-Simulink Converter  PhysicalDomain=network_engine_domain  SubClassName=ps_output  LeftPortType=input  RightPortType=output  PseudoPeriodic=off  Frequencies=[]  Unit=1  AffineConversion=off
  + : PMIOPort  Port=1  Side=Left
  - : PMIOPort  Port=2  Side=Right
  i : Outport
  wires:
  PS-Simulink Converter/1 -> i/1
  connections:
  PS-Simulink Converter/LConn1 -- Current Sensor/RConn1
  Current Sensor/RConn2 -- -/RConn1
  Current Sensor/LConn1 -- +/RConn1

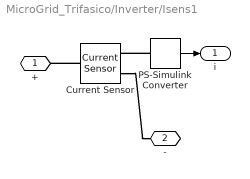
== system MicroGrid_Trifasico/Inverter/Isens1 ==
  Current Sensor : fl_lib/Electrical/Electrical Sensors/Current Sensor
  PS-Simulink Converter : nesl_utility/PS-Simulink Converter  PhysicalDomain=network_engine_domain  SubClassName=ps_output  LeftPortType=input  RightPortType=output  PseudoPeriodic=off  Frequencies=[]  Unit=1  AffineConversion=off
  + : PMIOPort  Port=1  Side=Left
  - : PMIOPort  Port=2  Side=Right
  i : Outport
  wires:
  PS-Simulink Converter/1 -> i/1
  connections:
  Current Sensor/LConn1 -- +/RConn1
  Current Sensor/RConn2 -- -/RConn1
  PS-Simulink Converter/LConn1 -- Current Sensor/RConn1

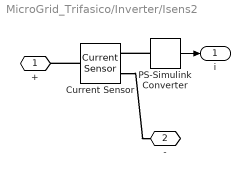
== system MicroGrid_Trifasico/Inverter/Isens2 ==
  Current Sensor : fl_lib/Electrical/Electrical Sensors/Current Sensor
  PS-Simulink Converter : nesl_utility/PS-Simulink Converter  PhysicalDomain=network_engine_domain  SubClassName=ps_output  LeftPortType=input  RightPortType=output  PseudoPeriodic=off  Frequencies=[]  Unit=1  AffineConversion=off
  + : PMIOPort  Port=1  Side=Left
  - : PMIOPort  Port=2  Side=Right
  i : Outport
  wires:
  PS-Simulink Converter/1 -> i/1
  connections:
  PS-Simulink Converter/LConn1 -- Current Sensor/RConn1
  Current Sensor/RConn2 -- -/RConn1
  Current Sensor/LConn1 -- +/RConn1

== system MicroGrid_Trifasico/Inverter/Steper1 ==
  In1 : Inport
  Product : Product
  Step : Step  Time=st_time3  SampleTime=0
  Out1 : Outport
  wires:
  Step/1 -> Product/2
  In1/1 -> Product/1
  Product/1 -> Out1/1

== system MicroGrid_Trifasico/Inverter/Steper2 ==
  In1 : Inport
  Product : Product
  Step : Step  Time=st_time3  SampleTime=0
  Out1 : Outport
  wires:
  Product/1 -> Out1/1
  In1/1 -> Product/1
  Step/1 -> Product/2

== system MicroGrid_Trifasico/Inverter/Steper3 ==
  In1 : Inport
  Product : Product
  Step : Step  Time=st_time3  SampleTime=0
  Out1 : Outport
  wires:
  Product/1 -> Out1/1
  In1/1 -> Product/1
  Step/1 -> Product/2

== system MicroGrid_Trifasico/Inverter/Steper4 ==
  In1 : Inport
  Product : Product
  Step : Step  Time=st_time3  SampleTime=0
  Out1 : Outport
  wires:
  Step/1 -> Product/2
  In1/1 -> Product/1
  Product/1 -> Out1/1

== system MicroGrid_Trifasico/Inverter/Steper5 ==
  In1 : Inport
  Product : Product
  Step : Step  Time=st_time3  SampleTime=0
  Out1 : Outport
  wires:
  Product/1 -> Out1/1
  In1/1 -> Product/1
  Step/1 -> Product/2

== system MicroGrid_Trifasico/Inverter/Steper6 ==
  In1 : Inport
  Product : Product
  Step : Step  Time=st_time3  SampleTime=0
  Out1 : Outport
  wires:
  Step/1 -> Product/2
  In1/1 -> Product/1
  Product/1 -> Out1/1

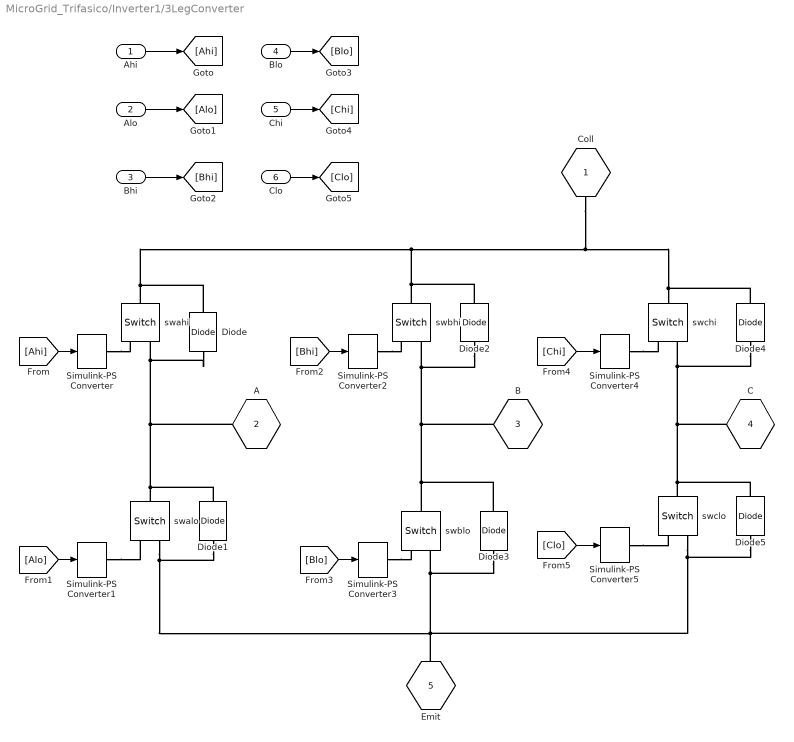
== system MicroGrid_Trifasico/Inverter1/3LegConverter ==
  Ahi : Inport
  Alo : Inport  Port=2
  Bhi : Inport  Port=3
  Blo : Inport  Port=4
  Chi : Inport  Port=5
  Clo : Inport  Port=6
  Diode{,1..5} (6 alike) : fl_lib/Electrical/Electrical Elements/Diode  Vf=0.6 V  Ron=0.3 Ohm  Goff=1e-8 1/Ohm  i_specify=off  i_priority=None  i=0 A  i_nominal_specify=off  i_nominal_unit=A  i_nominal_value=1  v_specify=off  v_priority=None  v=0 V  v_nominal_specify=off  v_nominal_unit=V  v_nominal_value=1
  Simulink-PS Converter{,1..5} (6 alike) : nesl_utility/Simulink-PS Converter  PhysicalDomain=network_engine_domain  SubClassName=ps_input  LeftPortType=input  RightPortType=output  PseudoPeriodic=off  Frequencies=[]  NoiseDistribution=none  NoiseParameters=[]  Unit=1  AffineConversion=off  FilteringAndDerivatives=zero  SimscapeFilterOrder=1  InputFilterTimeConstant=0.001  UdotUserProvided=1
  swahi : fl_lib/Electrical/Electrical Elements/Switch  R_closed=0.01 Ohm  G_open=1e-8 1/Ohm  Threshold=2  i_specify=off  i_priority=None  i=0 A  i_nominal_specify=off  i_nominal_unit=A  i_nominal_value=1  v_specify=off  v_priority=None  v=0 V  v_nominal_specify=off  v_nominal_unit=V  v_nominal_value=1
      settings: SourceProductName=Simscape
  swalo : fl_lib/Electrical/Electrical Elements/Switch  R_closed=0.01 Ohm  G_open=1e-8 1/Ohm  Threshold=2  i_specify=off  i_priority=None  i=0 A  i_nominal_specify=off  i_nominal_unit=A  i_nominal_value=1  v_specify=off  v_priority=None  v=0 V  v_nominal_specify=off  v_nominal_unit=V  v_nominal_value=1
      settings: SourceProductName=Simscape
  swbhi : fl_lib/Electrical/Electrical Elements/Switch  R_closed=0.01 Ohm  G_open=1e-8 1/Ohm  Threshold=2  i_specify=off  i_priority=None  i=0 A  i_nominal_specify=off  i_nominal_unit=A  i_nominal_value=1  v_specify=off  v_priority=None  v=0 V  v_nominal_specify=off  v_nominal_unit=V  v_nominal_value=1
      settings: SourceProductName=Simscape
  swblo : fl_lib/Electrical/Electrical Elements/Switch  R_closed=0.01 Ohm  G_open=1e-8 1/Ohm  Threshold=2  i_specify=off  i_priority=None  i=0 A  i_nominal_specify=off  i_nominal_unit=A  i_nominal_value=1  v_specify=off  v_priority=None  v=0 V  v_nominal_specify=off  v_nominal_unit=V  v_nominal_value=1
      settings: SourceProductName=Simscape
  swchi : fl_lib/Electrical/Electrical Elements/Switch  R_closed=0.01 Ohm  G_open=1e-8 1/Ohm  Threshold=2  i_specify=off  i_priority=None  i=0 A  i_nominal_specify=off  i_nominal_unit=A  i_nominal_value=1  v_specify=off  v_priority=None  v=0 V  v_nominal_specify=off  v_nominal_unit=V  v_nominal_value=1
      settings: SourceProductName=Simscape
  swclo : fl_lib/Electrical/Electrical Elements/Switch  R_closed=0.01 Ohm  G_open=1e-8 1/Ohm  Threshold=2  i_specify=off  i_priority=None  i=0 A  i_nominal_specify=off  i_nominal_unit=A  i_nominal_value=1  v_specify=off  v_priority=None  v=0 V  v_nominal_specify=off  v_nominal_unit=V  v_nominal_value=1
      settings: SourceProductName=Simscape
  Coll : PMIOPort  Port=1  Side=Right
  A : PMIOPort  Port=2  Side=Right
  B : PMIOPort  Port=3  Side=Right
  C : PMIOPort  Port=4  Side=Right
  Emit : PMIOPort  Port=5  Side=Right
  wires:
  Chi/1 -> [Chi]
  Blo/1 -> [Blo]
  [Chi] -> Simulink-PS Converter4/1
  Ahi/1 -> [Ahi]
  [Bhi] -> Simulink-PS Converter2/1
  Bhi/1 -> [Bhi]
  [Clo] -> Simulink-PS Converter5/1
  [Blo] -> Simulink-PS Converter3/1
  Alo/1 -> [Alo]
  Clo/1 -> [Clo]
  [Ahi] -> Simulink-PS Converter/1
  [Alo] -> Simulink-PS Converter1/1
  connections:
  swchi/RConn2 -- Diode4/LConn1 -- C/RConn1 -- Diode5/RConn1 -- swclo/LConn1
  swchi/LConn1 -- Diode4/RConn1 -- Coll/RConn1 -- swbhi/LConn1 -- Diode2/RConn1 -- Diode/RConn1 -- swahi/LConn1
  Diode1/RConn1 -- swahi/RConn2 -- Diode/LConn1 -- A/RConn1 -- swalo/LConn1
  Simulink-PS Converter1/RConn1 -- swalo/RConn1
  Simulink-PS Converter2/RConn1 -- swbhi/RConn1
  Simulink-PS Converter3/RConn1 -- swblo/RConn1
  swbhi/RConn2 -- Diode2/LConn1 -- B/RConn1 -- Diode3/RConn1 -- swblo/LConn1
  Simulink-PS Converter/RConn1 -- swahi/RConn1
  Simulink-PS Converter5/RConn1 -- swclo/RConn1
  Simulink-PS Converter4/RConn1 -- swchi/RConn1
  Diode1/LConn1 -- swclo/RConn2 -- Diode5/LConn1 -- Emit/RConn1 -- swblo/RConn2 -- Diode3/LConn1 -- swalo/RConn2

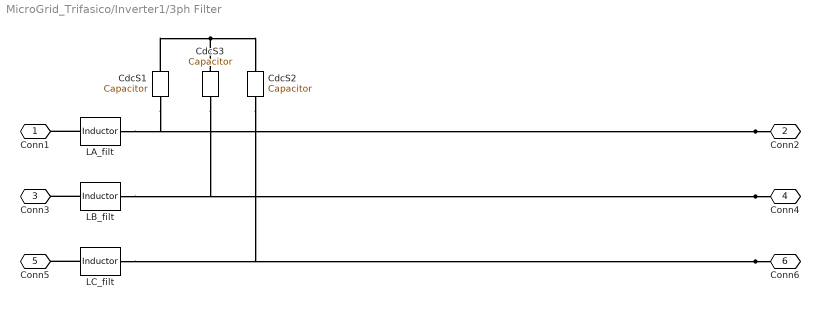
== system MicroGrid_Trifasico/Inverter1/3ph Filter ==
  CdcS1 : fl_lib/Electrical/Electrical Elements/Capacitor  c=3.5 uF  r=1e-6 Ohm  g=0 1/Ohm  i_specify=off  i_priority=None  i=0 A  i_nominal_specify=off  i_nominal_unit=A  i_nominal_value=1  v_specify=off  v_priority=None  v=0 V  v_nominal_specify=off  v_nominal_unit=V  v_nominal_value=1  vc_specify=on  vc_priority=High  vc=0 V  vc_nominal_specify=off  vc_nominal_unit=V  vc_nominal_value=1
  CdcS2 : fl_lib/Electrical/Electrical Elements/Capacitor  c=3.5 uF  r=1e-6 Ohm  g=0 1/Ohm  i_specify=off  i_priority=None  i=0 A  i_nominal_specify=off  i_nominal_unit=A  i_nominal_value=1  v_specify=off  v_priority=None  v=0 V  v_nominal_specify=off  v_nominal_unit=V  v_nominal_value=1  vc_specify=on  vc_priority=High  vc=0 V  vc_nominal_specify=off  vc_nominal_unit=V  vc_nominal_value=1
  CdcS3 : fl_lib/Electrical/Electrical Elements/Capacitor  c=3.5 uF  r=1e-6 Ohm  g=0 1/Ohm  i_specify=off  i_priority=None  i=0 A  i_nominal_specify=off  i_nominal_unit=A  i_nominal_value=1  v_specify=off  v_priority=None  v=0 V  v_nominal_specify=off  v_nominal_unit=V  v_nominal_value=1  vc_specify=on  vc_priority=High  vc=0 V  vc_nominal_specify=off  vc_nominal_unit=V  vc_nominal_value=1
  LA_filt : fl_lib/Electrical/Electrical Elements/Inductor  l=6.2 mH  r=0.1 Ohm  g=1e-6 1/Ohm  i_specify=off  i_priority=None  i=0 A  i_nominal_specify=off  i_nominal_unit=A  i_nominal_value=1  v_specify=off  v_priority=None  v=0 V  v_nominal_specify=off  v_nominal_unit=V  v_nominal_value=1  i_L_specify=on  i_L_priority=High  i_L=0 A  i_L_nominal_specify=off  i_L_nominal_unit=A  i_L_nominal_value=1
  LB_filt : fl_lib/Electrical/Electrical Elements/Inductor  l=6.2 mH  r=2 Ohm  g=1e-6 1/Ohm  i_specify=off  i_priority=None  i=0 A  i_nominal_specify=off  i_nominal_unit=A  i_nominal_value=1  v_specify=off  v_priority=None  v=0 V  v_nominal_specify=off  v_nominal_unit=V  v_nominal_value=1  i_L_specify=on  i_L_priority=High  i_L=0 A  i_L_nominal_specify=off  i_L_nominal_unit=A  i_L_nominal_value=1
  LC_filt : fl_lib/Electrical/Electrical Elements/Inductor  l=6.2 mH  r=2 Ohm  g=1e-6 1/Ohm  i_specify=off  i_priority=None  i=0 A  i_nominal_specify=off  i_nominal_unit=A  i_nominal_value=1  v_specify=off  v_priority=None  v=0 V  v_nominal_specify=off  v_nominal_unit=V  v_nominal_value=1  i_L_specify=on  i_L_priority=High  i_L=0 A  i_L_nominal_specify=off  i_L_nominal_unit=A  i_L_nominal_value=1
  Conn1 : PMIOPort  Port=1  Side=Left
  Conn2 : PMIOPort  Port=2  Side=Right
  Conn3 : PMIOPort  Port=3  Side=Left
  Conn4 : PMIOPort  Port=4  Side=Right
  Conn5 : PMIOPort  Port=5  Side=Left
  Conn6 : PMIOPort  Port=6  Side=Right
  connections:
  LB_filt/LConn1 -- Conn3/RConn1
  LA_filt/LConn1 -- Conn1/RConn1
  LC_filt/LConn1 -- Conn5/RConn1
  Conn6/RConn1 -- CdcS2/RConn1 -- LC_filt/RConn1
  Conn4/RConn1 -- CdcS3/RConn1 -- LB_filt/RConn1
  CdcS1/LConn1 -- CdcS2/LConn1 -- CdcS3/LConn1
  Conn2/RConn1 -- CdcS1/RConn1 -- LA_filt/RConn1

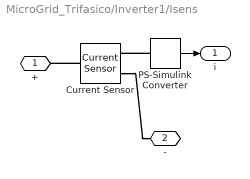
== system MicroGrid_Trifasico/Inverter1/Isens ==
  Current Sensor : fl_lib/Electrical/Electrical Sensors/Current Sensor
  PS-Simulink Converter : nesl_utility/PS-Simulink Converter  PhysicalDomain=network_engine_domain  SubClassName=ps_output  LeftPortType=input  RightPortType=output  PseudoPeriodic=off  Frequencies=[]  Unit=1  AffineConversion=off
  + : PMIOPort  Port=1  Side=Left
  - : PMIOPort  Port=2  Side=Right
  i : Outport
  wires:
  PS-Simulink Converter/1 -> i/1
  connections:
  Current Sensor/LConn1 -- +/RConn1
  Current Sensor/RConn2 -- -/RConn1
  PS-Simulink Converter/LConn1 -- Current Sensor/RConn1

== system MicroGrid_Trifasico/Inverter1/Isens1 ==
  Current Sensor : fl_lib/Electrical/Electrical Sensors/Current Sensor
  PS-Simulink Converter : nesl_utility/PS-Simulink Converter  PhysicalDomain=network_engine_domain  SubClassName=ps_output  LeftPortType=input  RightPortType=output  PseudoPeriodic=off  Frequencies=[]  Unit=1  AffineConversion=off
  + : PMIOPort  Port=1  Side=Left
  - : PMIOPort  Port=2  Side=Right
  i : Outport
  wires:
  PS-Simulink Converter/1 -> i/1
  connections:
  PS-Simulink Converter/LConn1 -- Current Sensor/RConn1
  Current Sensor/RConn2 -- -/RConn1
  Current Sensor/LConn1 -- +/RConn1

== system MicroGrid_Trifasico/Inverter1/Isens2 ==
  Current Sensor : fl_lib/Electrical/Electrical Sensors/Current Sensor
  PS-Simulink Converter : nesl_utility/PS-Simulink Converter  PhysicalDomain=network_engine_domain  SubClassName=ps_output  LeftPortType=input  RightPortType=output  PseudoPeriodic=off  Frequencies=[]  Unit=1  AffineConversion=off
  + : PMIOPort  Port=1  Side=Left
  - : PMIOPort  Port=2  Side=Right
  i : Outport
  wires:
  PS-Simulink Converter/1 -> i/1
  connections:
  Current Sensor/LConn1 -- +/RConn1
  Current Sensor/RConn2 -- -/RConn1
  PS-Simulink Converter/LConn1 -- Current Sensor/RConn1

== system MicroGrid_Trifasico/Inverter1/Steper1 ==
  In1 : Inport
  Product : Product
  Step : Step  Time=st_time3  SampleTime=0
  Out1 : Outport
  wires:
  Product/1 -> Out1/1
  In1/1 -> Product/1
  Step/1 -> Product/2

== system MicroGrid_Trifasico/Inverter1/Steper2 ==
  In1 : Inport
  Product : Product
  Step : Step  Time=st_time3  SampleTime=0
  Out1 : Outport
  wires:
  Step/1 -> Product/2
  In1/1 -> Product/1
  Product/1 -> Out1/1

== system MicroGrid_Trifasico/Inverter1/Steper3 ==
  In1 : Inport
  Product : Product
  Step : Step  Time=st_time3  SampleTime=0
  Out1 : Outport
  wires:
  Step/1 -> Product/2
  In1/1 -> Product/1
  Product/1 -> Out1/1

== system MicroGrid_Trifasico/Inverter1/Steper4 ==
  In1 : Inport
  Product : Product
  Step : Step  Time=st_time3  SampleTime=0
  Out1 : Outport
  wires:
  Product/1 -> Out1/1
  In1/1 -> Product/1
  Step/1 -> Product/2

== system MicroGrid_Trifasico/Inverter1/Steper5 ==
  In1 : Inport
  Product : Product
  Step : Step  Time=st_time3  SampleTime=0
  Out1 : Outport
  wires:
  Step/1 -> Product/2
  In1/1 -> Product/1
  Product/1 -> Out1/1

== system MicroGrid_Trifasico/Inverter1/Steper6 ==
  In1 : Inport
  Product : Product
  Step : Step  Time=st_time3  SampleTime=0
  Out1 : Outport
  wires:
  Product/1 -> Out1/1
  In1/1 -> Product/1
  Step/1 -> Product/2

== matlab function MicroGrid_Trifasico/Inverter/not_pwm1 ==
  data: u input; y output
function y = fcn(u)
%#codegen

if(u==0 || u<0)
    a=5;
else
    a=0;
end;

y = a;

== matlab function MicroGrid_Trifasico/Inverter/not_pwm ==
  data: u input; y output
function y = fcn(u)
%#codegen

if(u==0 || u<0)
    a=15;
else
    a=0;
end;

y = a;

== matlab function MicroGrid_Trifasico/Inverter/not_pwm2 ==
  data: u input; y output
function y = fcn(u)
%#codegen

if(u==0 || u<0)
    a=5;
else
    a=0;
end;

y = a;

== matlab function MicroGrid_Trifasico/Inverter1/not_pwm ==
  data: u input; y output
function y = fcn(u)
%#codegen

if(u==0 || u<0)
    a=15;
else
    a=0;
end;

y = a;

== matlab function MicroGrid_Trifasico/Inverter1/not_pwm1 ==
  data: u input; y output
function y = fcn(u)
%#codegen

if(u==0 || u<0)
    a=5;
else
    a=0;
end;

y = a;

== matlab function MicroGrid_Trifasico/Inverter1/not_pwm2 ==
  data: u input; y output
function y = fcn(u)
%#codegen

if(u==0 || u<0)
    a=5;
else
    a=0;
end;

y = a;
